simulink library "NullAircraftEstimateBus"  (R2018b)
settings: Solver=VariableStepAuto  StartTime=0.0  StopTime=10.0  RelTol=1e-3
libraries: signalsLib x3
settings Model: Creator=RA24876  LastModifiedBy=RA24876
settings SFSimCC: SimUseLocalCustomCode=off
settings RTWCC: RTWUseLocalCustomCode=off
settings CodeAppCC: StateflowObjectComments=on

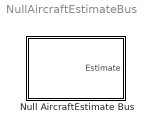
== system NullAircraftEstimateBus ==
  Null AircraftEstimate Bus : Subsystem  mask(Null AircraftEstimate Bus){}
      mask help: Creates an AircraftEstimate bus signal with all null values. Assign values to elements with a Bus Assignment block.

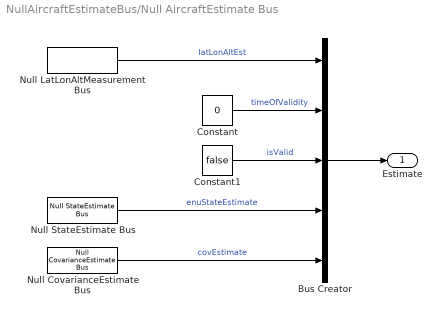
== system NullAircraftEstimateBus/Null AircraftEstimate Bus ==
  Bus Creator : BusCreator  Inputs='latLonAltEst','timeOfValidity','isValid','enuStateEstimate','covEstimate'
  Constant : Constant  Value=0
  Constant1 : Constant  Value=false  OutDataTypeStr=boolean
  Null CovarianceEstimate Bus : signalsLib/Signals/Bus Constructors/Null CovarianceEstimate Bus
      settings: SourceProductName=CASSATTv6: Signals Library
  Null LatLonAltMeasurement Bus : signalsLib/Signals/Bus Constructors/Null LatLonAltMeasurement Bus
      settings: SourceProductName=CASSATTv6: Signals Library
  Null StateEstimate Bus : signalsLib/Signals/Bus Constructors/Null StateEstimate Bus
      settings: SourceProductName=CASSATTv6: Signals Library
  Estimate : Outport  OutDataTypeStr=Bus: AircraftEstimate
  wires:
  Null CovarianceEstimate Bus/1 -> Bus Creator/5  "covEstimate"
  Constant1/1 -> Bus Creator/3  "isValid"
  Bus Creator/1 -> Estimate/1
  Constant/1 -> Bus Creator/2  "timeOfValidity"
  Null StateEstimate Bus/1 -> Bus Creator/4  "enuStateEstimate"
  Null LatLonAltMeasurement Bus/1 -> Bus Creator/1  "latLonAltEst"
